simulink model "car_sim2"  (R2013b)
settings: Solver=ode4  StartTime=0.0  StopTime=10  FixedStep=0.005  RelTol=1e-3
values from neighbouring files (symbols this model uses):
  ALC = A-L*C    [car.m]
  B = [1 ; 0]    [car.m]
  L = place(A', C', p)'    [car.m]
libraries: simulink x2
settings Model: Creator=ShengChieh  LastModifiedBy=ShengChieh
settings DataIOCC: LimitDataPoints=off

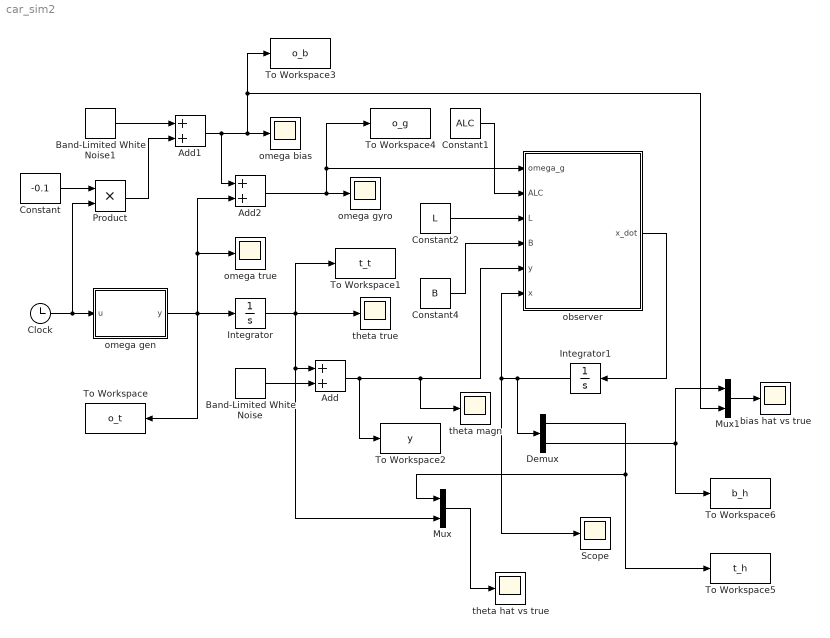
== system car_sim2 ==
  Add : Sum
  Add1 : Sum
  Add2 : Sum
  Band-Limited White Noise : simulink/Sources/Band-Limited White Noise  Cov=[0.00015]  Ts=0.005  seed=[23341]
  Band-Limited White Noise1 : simulink/Sources/Band-Limited White Noise  Cov=[0.0001]  Ts=0.005  seed=[23341]
  Clock : Clock
  Constant : Constant  Value=-0.1
  Constant1 : Constant  Value=ALC
  Constant2 : Constant  Value=L
  Constant4 : Constant  Value=B
  Demux : Demux  Outputs=2
  Integrator : Integrator
  Integrator1 : Integrator  InitialCondition=[0;0]
  Mux : Mux  Inputs=2
  Mux1 : Mux  Inputs=2
  Product : Product
  Scope : Scope
      settings: SaveName=ScopeData5
  To Workspace : ToWorkspace  VariableName=o_t  SampleTime=-1
  To Workspace1 : ToWorkspace  VariableName=t_t  SampleTime=-1
  To Workspace2 : ToWorkspace  VariableName=y  SampleTime=-1
  To Workspace3 : ToWorkspace  VariableName=o_b  SampleTime=-1
  To Workspace4 : ToWorkspace  VariableName=o_g  SampleTime=-1
  To Workspace5 : ToWorkspace  VariableName=t_h  SampleTime=-1
  To Workspace6 : ToWorkspace  VariableName=b_h  SampleTime=-1
  bias hat vs true : Scope
      settings: SaveName=ScopeData7
  observer : MATLAB Function  TreatAsAtomicUnit=on
  omega bias : Scope
  omega gen : MATLAB Function  TreatAsAtomicUnit=on
  omega gyro : Scope
      settings: SaveName=ScopeData4
  omega true : Scope
  theta hat vs true : Scope
      settings: SaveName=ScopeData6
  theta magn : Scope
      settings: SaveName=ScopeData3
  theta true : Scope
      settings: SaveName=ScopeData2
  wires:
  Clock/1 -> Product/2, omega gen/1(u)
  omega gen/1(y) -> To Workspace/1, Integrator/1, Add2/2, omega true/1
  Integrator/1 -> To Workspace1/1, Mux/2, Add/1, theta true/1
  Band-Limited White Noise/1 -> Add/2
  Add/1 -> observer/5(y), theta magn/1, To Workspace2/1
  Constant/1 -> Product/1
  Band-Limited White Noise1/1 -> Add1/1
  Product/1 -> Add1/2
  Add1/1 -> To Workspace3/1, Mux1/2, omega bias/1, Add2/1
  Add2/1 -> To Workspace4/1, observer/1(omega_g), omega gyro/1
  observer/1(x_dot) -> Integrator1/1
  Integrator1/1 -> Demux/1, Scope/1, observer/6(x)
  Constant1/1 -> observer/2(ALC)
  Constant2/1 -> observer/3(L)
  Constant4/1 -> observer/4(B)
  Demux/1 -> To Workspace5/1, Mux/1
  Mux/1 -> theta hat vs true/1
  Mux1/1 -> bias hat vs true/1
  Demux/2 -> To Workspace6/1, Mux1/1

== matlab function car_sim2/observer ==
  data: omega_g input; ALC input; L input; B input; y input; x input; x_dot output
function x_dot = fcn(omega_g,ALC,L,B,y,x)

x_dot = ALC*x + B*omega_g + L*y;

== matlab function car_sim2/omega gen ==
  data: u input; y output
function y = fcn(u)

y = 1*sqrt(u)-5*sin(2*u)+0.002*u-0.05*u^2;
